simulink model "BaseEngineController_LS_112"  (Simulink 7.7)
settings: Solver=FixedStepDiscrete  StartTime=0.0  StopTime=10.0  RelTol=1e-3
PreLoadFcn:
  | try, eval([bdroot '_setup']); catch, eval('model_setup', ''); end
InitFcn:
  | try, eval([bdroot '_setup']); catch, eval('model_setup', ''); end
undefined symbols (not defined in the file): ECM, H1, H2, High, motohawk_build_version, motohawk_trunc_name, motohawk_vardec_config_group, motohawk_vardec_path, True, xD
libraries: MotoHawk_lib x1417, motohawk_control_primitives_lib x183, motohawk_engine_lib x32, simulink x21, motohawk_annotations_lib x9, AutoDoc_lib x8, simulink_extras x4, motohawk_ccp_examples_lib x1, motohawk_control_primitives_motoshare_lib x1
(part 16 of 27)

== system BaseEngineController_LS_112/Foreground/Control/VirtualSensors/AirCalcs/Speed Density - MAP Referenced - Adaptive ==
  note: mdot = rho V A = rho Q = (p/RT) (ve Vcyl) (Neng Ncyl / 60 NRPC )
  BARO [kPa] : Inport
  MAP [kPa] : Inport  Port=2
  RPM : Inport  Port=3
  IAT [C] : Inport  Port=4
  MAF_Sensor [g/s] : Inport  Port=5
  IAT17Idx : Inport  Port=6
  RPMIdx : Inport  Port=7
  SSEngOpr [bool] : Inport  Port=8
  ECT09Idx : Inport  Port=9
  ECT [C] : Inport  Port=10
  TimeAfterRun [S] : Inport  Port=11
  EngState : Inport  Port=12
  Adapt VolEff Map : Subsystem
  C to K1 : Subsystem
      mask Display: disp('to')
  Compare To Constant : simulink/Logic and Bit Operations/Compare To Constant  SystemSampleTime=-1  relop===  const=3  LogicOutDataTypeMode=boolean
  Cylinder Swept Volume [cm3]1 : MotoHawk_lib/Data Storage Blocks/motohawk_data_def  nam='CylSweptVol'  container_nam=''  data=373.5  typ=double  struct_nam='MyStruct'  storage=Constant  outputRef=off  use_vardec=on  window=Calibration  read_level=1  write_level=1  ovr_cals=on  view_as=Number  enum_struct={'Disabled', 'Enabled'}  vector_style=Wide Row  use_help_units=off  help='Cylinder swept volume for a single cylinder.'  units='cm3'  use_header_enum=off  row_header_enum={}  col_header_enum={}  use_min_max=off  min_val=0  max_val=inf  use_precision=on  precision=''  gain=1  offset=0  exp=1  use_mototune_group=on  mototune_group=motohawk_vardec_path(gcb)  eval_name=CylSweptVol  data_stores=motohawk_sfun_data_def_data_stores  struct_instances=motohawk_sfun_data_def_struct_instances  vardecs=motohawk_sfun_data_def_vardecs
  Cylinder Swept Volume [cm3] : MotoHawk_lib/Data Storage Blocks/motohawk_data_read  source=Lookup By Name  structure=Scalar  operation=Read scalar from location by index  sz_vec=-1  sz_row=-1  sz_col=-1  typ=double  nam='CylSweptVol'  checkNull=on  struct_inst_name='Struct1'  struct_nam='MyStruct'
  Data Type Conversion : DataTypeConversion  SaturateOnIntegerOverflow=on  RndMeth=Zero
  Gas Const [J/kg-K] : Constant  Value=287  OutDataTypeStr=Inherit: Inherit via back propagation
  Logical Operator : Logic  Inputs=6
  Logical Operator1 : Logic  Operator=NOT  AllPortsSameDT=off  OutDataTypeStr=boolean
  Model Air Mass Flow Rate : Product  Inputs=**  SaturateOnIntegerOverflow=on  InputSameDT=on  OutDataTypeStr=Inherit: Same as first input
  Multiport Switch : MultiPortSwitch  DataPortOrder=Zero-based contiguous  Inputs=2  zeroidx=on  SaturateOnIntegerOverflow=on  InputSameDT=on
  Nominal Air Flow Rate : Product  Inputs=******///  SaturateOnIntegerOverflow=on  InputSameDT=on  OutDataTypeStr=Inherit: Same as first input
  Number of Combustion Events Per Revolution : MotoHawk_lib/Data Storage Blocks/motohawk_data_read  source=Lookup By Name  structure=Scalar  operation=Read scalar from location by index  sz_vec=-1  sz_row=-1  sz_col=-1  typ=uint8  nam='CombEventsPerRev'  checkNull=on  struct_inst_name='Struct1'  struct_nam='MyStruct'
  Number of Combustion Events Per Revolution1 : MotoHawk_lib/Data Storage Blocks/motohawk_data_def  nam='CombEventsPerRev'  container_nam=''  data=1  typ=uint8  struct_nam='MyStruct'  storage=Constant  outputRef=off  use_vardec=on  window=Calibration  read_level=1  write_level=1  ovr_cals=on  view_as=Number  enum_struct={'Disabled', 'Enabled'}  vector_style=Wide Row  use_help_units=on  help='Number of conbustion events per engine revolution. For example, for a four-stroke, eight cylinder engine the value would be 4.'  units=''  use_header_enum=off  row_header_enum={}  col_header_enum={}  use_min_max=on  min_val=.5  max_val=inf  use_precision=off  precision=''  gain=1  offset=0  exp=1  use_mototune_group=on  mototune_group=motohawk_vardec_path(gcb)  eval_name=CombEventsPerRev  data_stores=motohawk_sfun_data_def_data_stores  struct_instances=motohawk_sfun_data_def_struct_instances  vardecs=motohawk_sfun_data_def_vardecs
  Relational Operator1 : RelationalOperator  InputSameDT=on
  Relational Operator2 : RelationalOperator  InputSameDT=on
  Sum : Sum  Inputs=|++
  Units Equivalency Factor : Constant  Value=60  OutDataTypeStr=Inherit: Inherit via back propagation
  motohawk_calibration : MotoHawk_lib/Calibration & Probing Blocks/motohawk_calibration  nam='VEAdaptEnable'  val=0  storage=Calibration  show_more=on  name_source=Use Parameter  data_type=boolean  read_level=1  write_level=1  ovr_cals=on  view_as=Enumeration  enum_struct={'Disabled', 'Enabled'}  vector_style=Wide Row  use_help_units=on  help='Determines whether the Volumetric Efficiency map will be adapted using the MAF sensor'  units='bool'  use_header_enum=off  row_header_enum={}  col_header_enum={}  use_min_max=off  min_val=-inf  max_val=inf  use_precision=off  precision=''  gain=1  offset=0  exp=1  use_mototune_group=on  mototune_group=motohawk_vardec_path(gcb)
  motohawk_calibration1 : MotoHawk_lib/Calibration & Probing Blocks/motohawk_calibration  nam='MAF_Source'  val=0  storage=Calibration  show_more=on  name_source=Use Parameter  data_type=uint8  read_level=1  write_level=1  ovr_cals=on  view_as=Enumeration  enum_struct={'Model from MAP', 'Use MAF sensor directly'}  vector_style=Wide Row  use_help_units=on  help='Selects the source for the fueling algorithm'  units=''  use_header_enum=off  row_header_enum={}  col_header_enum={}  use_min_max=off  min_val=-inf  max_val=inf  use_precision=off  precision=''  gain=1  offset=0  exp=1  use_mototune_group=on  mototune_group=motohawk_vardec_path(gcb)
  motohawk_calibration2 : MotoHawk_lib/Calibration & Probing Blocks/motohawk_calibration  nam='VEAdaptTemp'  val=60  storage=Calibration  show_more=on  name_source=Use Parameter  data_type=Inherit from 'Default Value'  read_level=1  write_level=1  ovr_cals=on  view_as=Number  enum_struct={'Disabled', 'Enabled'}  vector_style=Wide Row  use_help_units=on  help='Engine Coolant Temp Must be higher than this to Adapt VE'  units='degC'  use_header_enum=off  row_header_enum={}  col_header_enum={}  use_min_max=on  min_val=-40  max_val=200  use_precision=off  precision=''  gain=1  offset=0  exp=1  use_mototune_group=on  mototune_group=motohawk_vardec_path(gcb)
  motohawk_calibration3 : MotoHawk_lib/Calibration & Probing Blocks/motohawk_calibration  nam='VEAdaptTime'  val=60  storage=Calibration  show_more=on  name_source=Use Parameter  data_type=Inherit from 'Default Value'  read_level=1  write_level=1  ovr_cals=on  view_as=Number  enum_struct={'Disabled', 'Enabled'}  vector_style=Wide Row  use_help_units=on  help='Engine Run Time must be greater than this to Adapt VE'  units='sec'  use_header_enum=off  row_header_enum={}  col_header_enum={}  use_min_max=on  min_val=0  max_val=200  use_precision=off  precision=''  gain=1  offset=0  exp=1  use_mototune_group=on  mototune_group=motohawk_vardec_path(gcb)
  motohawk_fault_action1 : MotoHawk_lib/Fault Management Blocks/motohawk_fault_action  nam='DisableVEAdapt'  output_status=on  eval_nam=DisableVEAdapt
  motohawk_interpolation_1d1 : MotoHawk_lib/Lookup Tables/motohawk_interpolation_1d  nam='VEBaroCorr'  table_data=[1 1 1 1 1 1 1 1 1]  show_more=on  data_type=Inherit from 'Table Data'  storage=NonAdaptive  read_level=1  write_level=1  ovr_cals=on  use_help=on  help='Vol Eff compensation based on BARO.'  units=''  use_min_max=on  min_val=-inf  max_val=inf  use_precision=on  precision=''  gain=1  offset=0  exp=1  use_links=off  prelookup_block=''  output_name=''  use_mototune_group=on  mototune_group=motohawk_vardec_path(gcb)
  motohawk_interpolation_2d : MotoHawk_lib/Lookup Tables/motohawk_interpolation_2d  nam='VolEff'  table_data=ones(17)  show_more=on  data_type=Inherit from 'Table Data'  storage=NonAdaptive  read_level=1  write_level=1  ovr_cals=on  use_help=on  help='Volumetric efficiency table for speed density mode'  units='%'  use_min_max=on  min_val=0  max_val=1000  use_precision=on  precision=''  gain=1  offset=0  exp=1  use_links=on  row_prelookup_block=''  col_prelookup_block=''  output_name=''  use_mototune_group=on  mototune_group=motohawk_vardec_path(gcb)
  motohawk_interpolation_2d1 : MotoHawk_lib/Lookup Tables/motohawk_interpolation_2d  nam='VETempCorr'  table_data=ones(17,9)  show_more=on  data_type=Inherit from 'Table Data'  storage=NonAdaptive  read_level=1  write_level=1  ovr_cals=on  use_help=on  help=''  units='%'  use_min_max=off  min_val=-inf  max_val=inf  use_precision=off  precision=''  gain=1  offset=0  exp=1  use_links=off  row_prelookup_block=''  col_prelookup_block=''  output_name=''  use_mototune_group=off  mototune_group=motohawk_vardec_path(gcb)
  motohawk_interpolation_2d2 : MotoHawk_lib/Lookup Tables/motohawk_interpolation_2d  nam='VolEffAdapt'  table_data=ones(17)  show_more=on  data_type=Inherit from 'Table Data'  storage=Adaptive - NonVolatile  read_level=1  write_level=1  ovr_cals=on  use_help=on  help='Volumetric efficiency adapt table'  units='%'  use_min_max=on  min_val=-1000  max_val=1000  use_precision=on  precision=''  gain=1  offset=0  exp=1  use_links=on  row_prelookup_block=''  col_prelookup_block=''  output_name=''  use_mototune_group=on  mototune_group=motohawk_vardec_path(gcb)
  motohawk_prelookup1 : MotoHawk_lib/Lookup Tables/motohawk_prelookup  nam='BARO09'  breakpoint_data=[60 70 75 80 85 90 95 98 100]  show_more=on  data_type=Inherit from 'Table Data'  storage=Constant  read_level=1  write_level=1  ovr_cals=on  use_help=on  help=''  units=''  use_min_max=off  min_val=-inf  max_val=inf  use_precision=on  precision=''  gain=1  offset=0  exp=1  use_links=on  input_name='BARO'  use_mototune_group=on  mototune_group=motohawk_vardec_path(gcb)
  motohawk_prelookup2 : MotoHawk_lib/Lookup Tables/motohawk_prelookup  nam='VEMap'  breakpoint_data=[1:17]  show_more=on  data_type=Inherit from 'Table Data'  storage=Constant  read_level=1  write_level=1  ovr_cals=on  use_help=on  help='Index of MAP for VE calculations'  units='kPa'  use_min_max=off  min_val=-inf  max_val=inf  use_precision=on  precision=''  gain=1  offset=0  exp=1  use_links=off  input_name=''  use_mototune_group=on  mototune_group=motohawk_vardec_path(gcb)
  motohawk_probe : MotoHawk_lib/Calibration & Probing Blocks/motohawk_probe  nam='VEModelMAF'  show_more=on  name_source=Use Parameter  read_level=1  view_as=Number  enum_struct={'Disabled', 'Enabled'}  vector_style=Wide Row  use_help_units=on  help='Air Mass Flow Rate - Port Total'  units='g/s'  use_header_enum=off  row_header_enum={}  col_header_enum={}  use_precision=off  precision=''  gain=1  offset=0  exp=1  use_mototune_group=on  mototune_group=motohawk_vardec_path(gcb)
  motohawk_probe1 : MotoHawk_lib/Calibration & Probing Blocks/motohawk_probe  nam='VEIdealMAF'  show_more=on  name_source=Use Parameter  read_level=1  view_as=Number  enum_struct={'Disabled', 'Enabled'}  vector_style=Wide Row  use_help_units=on  help='Air Mass Flow Rate - ideal'  units='g/s'  use_header_enum=off  row_header_enum={}  col_header_enum={}  use_precision=off  precision=''  gain=1  offset=0  exp=1  use_mototune_group=on  mototune_group=motohawk_vardec_path(gcb)
  motohawk_probe3 : MotoHawk_lib/Calibration & Probing Blocks/motohawk_probe  nam='MAFFinal'  show_more=on  name_source=Use Parameter  read_level=1  view_as=Number  enum_struct={'Disabled', 'Enabled'}  vector_style=Wide Row  use_help_units=on  help='Air mass flow rate at the intake manifold - Used by the fueling algorithm'  units='g/s'  use_header_enum=off  row_header_enum={}  col_header_enum={}  use_precision=off  precision=''  gain=1  offset=0  exp=1  use_mototune_group=on  mototune_group=motohawk_vardec_path(gcb)
  motohawk_probe4 : MotoHawk_lib/Calibration & Probing Blocks/motohawk_probe  nam='VEAdapting'  show_more=on  name_source=Use Parameter  read_level=1  view_as=Enumeration  enum_struct={'Not adapting', 'Adapting'}  vector_style=Wide Row  use_help_units=on  help='Indicates whether the volumetric efficiency map is currently being adjusted'  units=''  use_header_enum=off  row_header_enum={}  col_header_enum={}  use_precision=off  precision=''  gain=1  offset=0  exp=1  use_mototune_group=on  mototune_group=motohawk_vardec_path(gcb)
  motohawk_probe5 : MotoHawk_lib/Calibration & Probing Blocks/motohawk_probe  nam='VEFin'  show_more=on  name_source=Use Parameter  read_level=1  view_as=Number  enum_struct={'Disabled', 'Enabled'}  vector_style=Wide Row  use_help_units=on  help='Final volumentric efficiency after adapt table'  units='g/s'  use_header_enum=off  row_header_enum={}  col_header_enum={}  use_precision=off  precision=''  gain=1  offset=0  exp=1  use_mototune_group=on  mototune_group=motohawk_vardec_path(gcb)
  motohawk_probe6 : MotoHawk_lib/Calibration & Probing Blocks/motohawk_probe  nam='VEAdaptAmnt'  show_more=on  name_source=Use Parameter  read_level=1  view_as=Number  enum_struct={'Disabled', 'Enabled'}  vector_style=Wide Row  use_help_units=on  help='Volumetric efficiency adapt amount at the given speed and load'  units='%'  use_header_enum=off  row_header_enum={}  col_header_enum={}  use_precision=off  precision=''  gain=1  offset=0  exp=1  use_mototune_group=on  mototune_group=motohawk_vardec_path(gcb)
  MAF [g/s] : Outport
  wires:
  motohawk_calibration1/1 -> Multiport Switch/1
  Multiport Switch/1 -> motohawk_probe3/1, MAF [g/s]/1
  MAF_Sensor [g/s]/1 -> Multiport Switch/3, Adapt VolEff Map/1(MAFSens)
  RPMIdx/1 -> motohawk_interpolation_2d/2, motohawk_interpolation_2d2/2
  motohawk_prelookup2/1 -> motohawk_interpolation_2d/1, motohawk_interpolation_2d2/1
  Model Air Mass Flow Rate/1 -> motohawk_probe/1, Multiport Switch/2, Adapt VolEff Map/2(MAFSpdDensity)
  IAT [C]/1 -> C to K1/1(C)
  RPM/1 -> Nominal Air Flow Rate/1
  BARO [kPa]/1 -> motohawk_prelookup1/1
  MAP [kPa]/1 -> Nominal Air Flow Rate/2, motohawk_prelookup2/1
  motohawk_interpolation_2d1/1 -> Nominal Air Flow Rate/4
  Cylinder Swept Volume [cm3]/1 -> Nominal Air Flow Rate/5
  Number of Combustion Events Per Revolution/1 -> Data Type Conversion/1
  C to K1/1(K) -> Nominal Air Flow Rate/7
  Units Equivalency Factor/1 -> Nominal Air Flow Rate/8
  Gas Const [J/kg-K]/1 -> Nominal Air Flow Rate/9
  Nominal Air Flow Rate/1 -> Model Air Mass Flow Rate/2, motohawk_probe1/1
  Data Type Conversion/1 -> Nominal Air Flow Rate/6
  motohawk_prelookup1/1 -> motohawk_interpolation_1d1/1
  motohawk_interpolation_1d1/1 -> Nominal Air Flow Rate/3
  IAT17Idx/1 -> motohawk_interpolation_2d1/1
  ECT09Idx/1 -> motohawk_interpolation_2d1/2
  motohawk_fault_action1/1 -> Logical Operator1/1
  EngState/1 -> Compare To Constant/1
  Compare To Constant/1 -> Logical Operator/1
  Logical Operator1/1 -> Logical Operator/2
  SSEngOpr [bool]/1 -> Logical Operator/3
  ECT [C]/1 -> Relational Operator1/1
  Relational Operator1/1 -> Logical Operator/4
  Relational Operator2/1 -> Logical Operator/5
  motohawk_calibration2/1 -> Relational Operator1/2
  TimeAfterRun [S]/1 -> Relational Operator2/1
  motohawk_calibration3/1 -> Relational Operator2/2
  Logical Operator/1 -> Adapt VolEff Map/Enable, motohawk_probe4/1
  motohawk_calibration/1 -> Logical Operator/6
  motohawk_interpolation_2d/1 -> Sum/1
  motohawk_interpolation_2d2/1 -> Sum/2, motohawk_probe6/1
  Sum/1 -> Model Air Mass Flow Rate/1, Adapt VolEff Map/3(VE), motohawk_probe5/1

== system BaseEngineController_LS_112/Foreground/Control/VirtualSensors/FuelLevel/FuelLevelWrite ==
  FuelLevelFilt : Inport
  Enable : EnablePort
  motohawk_data_write : MotoHawk_lib/Data Storage Blocks/motohawk_data_write  source=Lookup By Name  structure=Scalar  operation=Write entire data structure at once  sz_vec=9  sz_row=2  sz_col=9  typ=double  nam='FuelLvl_NVM'  checkNull=on  write_read_only=off  struct_inst_name=''  struct_name='MyStruct'
  wires:
  FuelLevelFilt/1 -> motohawk_data_write/1

== system BaseEngineController_LS_112/Foreground/Control/VirtualSensors/FuelLevel/RefuelEvent ==
  FuelRaw : Inport
  TimeSinceKeyOn : Inport  Port=2
  Logical Operator : Logic  AllPortsSameDT=off  OutDataTypeStr=boolean
  Relational Operator : RelationalOperator  OutDataTypeStr=boolean
  Relational Operator1 : RelationalOperator  OutDataTypeStr=boolean
  Rising Edge : motohawk_control_primitives_lib/Rising Edge  SystemSampleTime=-1
  Sum : Sum  Inputs=|+-
  motohawk_calibration1 : MotoHawk_lib/Calibration & Probing Blocks/motohawk_calibration  nam='FuelLevl_KeyUpDiff'  val=5  storage=Calibration  show_more=on  name_source=Use Parameter  data_type=Inherit from 'Default Value'  read_level=1  write_level=1  ovr_cals=on  view_as=Number  enum_struct={'Disabled', 'Enabled'}  vector_style=Wide Row  use_help_units=on  help='Fuel level key up different for refuel event'  units='%'  use_header_enum=off  row_header_enum={}  col_header_enum={}  use_min_max=on  min_val=0  max_val=inf  use_precision=off  precision=''  gain=1  offset=0  exp=1  use_mototune_group=off  mototune_group=motohawk_vardec_path(gcb)
  motohawk_calibration10 : MotoHawk_lib/Calibration & Probing Blocks/motohawk_calibration  nam='FuelLevel_KeyUpDelay'  val=.2  storage=Calibration  show_more=on  name_source=Use Parameter  data_type=Inherit from 'Default Value'  read_level=1  write_level=1  ovr_cals=on  view_as=Number  enum_struct={'Disabled', 'Enabled'}  vector_style=Wide Row  use_help_units=on  help='Fuel level time from key on delay'  units='sec'  use_header_enum=off  row_header_enum={}  col_header_enum={}  use_min_max=on  min_val=0  max_val=inf  use_precision=off  precision=''  gain=1  offset=0  exp=1  use_mototune_group=off  mototune_group=motohawk_vardec_path(gcb)
  motohawk_data_read : MotoHawk_lib/Data Storage Blocks/motohawk_data_read  source=Lookup By Name  structure=Scalar  operation=Read scalar from location by index  sz_vec=4  sz_row=2  sz_col=3  typ=double  nam='FuelLvl_NVM'  checkNull=on  struct_inst_name='MyData'  struct_nam='MyStruct'
  motohawk_probe : MotoHawk_lib/Calibration & Probing Blocks/motohawk_probe  nam='FuelLevel_RefuelEvent'  show_more=off  name_source=Use Parameter  read_level=1  view_as=Number  enum_struct={'Disabled', 'Enabled'}  vector_style=Wide Row  use_help_units=off  help=''  units=''  use_header_enum=off  row_header_enum={}  col_header_enum={}  use_precision=off  precision=''  gain=1  offset=0  exp=1  use_mototune_group=off  mototune_group=motohawk_vardec_path(gcb)
  RefuelEvent : Outport
  RefuelEventDR : Outport  Port=2
  wires:
  TimeSinceKeyOn/1 -> Relational Operator/1
  motohawk_calibration10/1 -> Relational Operator/2
  Relational Operator/1 -> RefuelEventDR/1, Logical Operator/2
  FuelRaw/1 -> Sum/1
  motohawk_data_read/1 -> Sum/2
  Sum/1 -> Relational Operator1/1
  motohawk_calibration1/1 -> Relational Operator1/2
  Relational Operator1/1 -> Logical Operator/1
  Logical Operator/1 -> Rising Edge/1
  Rising Edge/1 -> RefuelEvent/1, motohawk_probe/1

== system BaseEngineController_LS_112/Foreground/Control/VirtualSensors/LoadBasedCalcs/Engine Steady-State Flag ==
  Load : Inport
  RPM : Inport  Port=2
  Abs : Abs  SaturateOnIntegerOverflow=on
  Abs1 : Abs  SaturateOnIntegerOverflow=on
  Constant : Constant  Value=0  OutDataTypeStr=Inherit: Inherit via back propagation
  Inc_DecFilterSelect1 : Subsystem  AncestorBlock=motohawk_control_primitives_lib/Inc_DecFilterSelect1  mask{nam='SSRPM', grp_dis=group, grp_cal=motohawk_vardec_config_group(group)}
      mask prompts: nam "Signal Name"; grp_dis "MotoTune Display Group"; grp_cal "MotoTune Calibration Group"
      mask Display:
      | patch([0 0 1 1], [0 0.075 0.075 0], [230/255 0/255 0/255])
      | patch([0 0 1 1], [0.025 0.05 0.05 0.025], [150/255 0/255 0/255])
      | patch([0 0 1 1], [0 0.025 0.025 0], [0/255 0/255 0/255])
      | 
      | disp('Increasing/Decreasing\nFiler Select');
  Inc_DecFilterSelect3 : Subsystem  AncestorBlock=motohawk_control_primitives_lib/Inc_DecFilterSelect1  mask{nam='SSLoad', grp_dis=group, grp_cal=motohawk_vardec_config_group(group)}
      mask prompts: nam "Signal Name"; grp_dis "MotoTune Display Group"; grp_cal "MotoTune Calibration Group"
      mask Display:
      | patch([0 0 1 1], [0 0.075 0.075 0], [230/255 0/255 0/255])
      | patch([0 0 1 1], [0.025 0.05 0.05 0.025], [150/255 0/255 0/255])
      | patch([0 0 1 1], [0 0.025 0.025 0], [0/255 0/255 0/255])
      | 
      | disp('Increasing/Decreasing\nFiler Select');
  Logical Operator : Logic  Inputs=3
  Relational Operator : RelationalOperator  Operator=<=  InputSameDT=on
  Relational Operator1 : RelationalOperator  Operator=<=  InputSameDT=on
  Relational Operator2 : RelationalOperator  Operator=>  ZeroCross=off  InputSameDT=on
  Steady-state RPM Tolerance [RPM] : MotoHawk_lib/Calibration & Probing Blocks/motohawk_calibration  nam='SSRPMTol'  val=600  storage=Calibration  show_more=on  name_source=Use Parameter  data_type=Inherit from 'Default Value'  read_level=1  write_level=1  ovr_cals=on  view_as=Number  enum_struct={'Disabled', 'Enabled'}  vector_style=Wide Row  use_help_units=on  help='Steady-State RPM Tolerance'  units='RPM'  use_header_enum=off  row_header_enum={}  col_header_enum={}  use_min_max=off  min_val=-inf  max_val=inf  use_precision=off  precision=''  gain=1  offset=0  exp=1  use_mototune_group=on  mototune_group=motohawk_vardec_path(gcb)
  Steady-state Torque Tolerance [N.m] : MotoHawk_lib/Calibration & Probing Blocks/motohawk_calibration  nam='SSLoadTol'  val=100  storage=Calibration  show_more=on  name_source=Use Parameter  data_type=Inherit from 'Default Value'  read_level=1  write_level=1  ovr_cals=on  view_as=Number  enum_struct={'Disabled', 'Enabled'}  vector_style=Wide Row  use_help_units=on  help='Steady-State Load Tolerance'  units=''  use_header_enum=off  row_header_enum={}  col_header_enum={}  use_min_max=off  min_val=-inf  max_val=inf  use_precision=off  precision=''  gain=1  offset=0  exp=1  use_mototune_group=on  mototune_group=motohawk_vardec_path(gcb)
  Sum : Sum  Inputs=+-|  SaturateOnIntegerOverflow=on  InputSameDT=on  OutDataTypeStr=Inherit: Same as first input
  Sum1 : Sum  Inputs=+-|  SaturateOnIntegerOverflow=on  InputSameDT=on  OutDataTypeStr=Inherit: Same as first input
  motohawk_probe : MotoHawk_lib/Calibration & Probing Blocks/motohawk_probe  nam='SSEngOpr'  show_more=on  name_source=Use Parameter  read_level=1  view_as=Enumeration  enum_struct={'Transient', 'Steady'}  vector_style=Wide Row  use_help_units=on  help='Steady-State Engine Operation'  units=''  use_header_enum=off  row_header_enum={}  col_header_enum={}  use_precision=off  precision=''  gain=1  offset=0  exp=1  use_mototune_group=on  mototune_group=motohawk_vardec_path(gcb)
  SSEngOpr [bool] : Outport
  wires:
  Steady-state RPM Tolerance [RPM]/1 -> Relational Operator1/2
  Steady-state Torque Tolerance [N.m]/1 -> Relational Operator/2
  Inc_DecFilterSelect1/1(Out) -> Sum1/2
  Logical Operator/1 -> SSEngOpr [bool]/1, motohawk_probe/1
  Abs1/1 -> Relational Operator1/1
  Sum1/1 -> Abs1/1
  Abs/1 -> Relational Operator/1
  Sum/1 -> Abs/1
  Inc_DecFilterSelect3/1(Out) -> Sum/2
  RPM/1 -> Sum1/1, Relational Operator2/1, Inc_DecFilterSelect1/1(In)
  Load/1 -> Sum/1, Inc_DecFilterSelect3/1(In)
  Relational Operator1/1 -> Logical Operator/1
  Relational Operator/1 -> Logical Operator/3
  Relational Operator2/1 -> Logical Operator/2
  Constant/1 -> Relational Operator2/2

== system BaseEngineController_LS_112/Foreground/Control/VirtualSensors/Raw Indexes/ACPres Index ==
  ACPres : Inport
  motohawk_prelookup : MotoHawk_lib/Lookup Tables/motohawk_prelookup  nam='ACPres05'  breakpoint_data=[1500 1750 2000 2250 2500]  show_more=on  data_type=Inherit from 'Table Data'  storage=Constant  read_level=1  write_level=1  ovr_cals=on  use_help=on  help='Index of AC system high side pressure'  units='kPa'  use_min_max=on  min_val=-150  max_val=10000  use_precision=on  precision=''  gain=1  offset=0  exp=1  use_links=off  input_name=''  use_mototune_group=on  mototune_group=motohawk_vardec_path(gcb)
  motohawk_prelookup1 : MotoHawk_lib/Lookup Tables/motohawk_prelookup  nam='ACPres07'  breakpoint_data=[1500 1750 2000 2250 2500 2500 2500]  show_more=on  data_type=Inherit from 'Table Data'  storage=Constant  read_level=1  write_level=1  ovr_cals=on  use_help=on  help='Index of AC system high side pressure'  units='kPa'  use_min_max=on  min_val=-150  max_val=10000  use_precision=on  precision=''  gain=1  offset=0  exp=1  use_links=off  input_name=''  use_mototune_group=on  mototune_group=motohawk_vardec_path(gcb)
  ACPres05Idx : Outport
  ACPres07Idx : Outport  Port=2
  wires:
  ACPres/1 -> motohawk_prelookup/1, motohawk_prelookup1/1
  motohawk_prelookup/1 -> ACPres05Idx/1
  motohawk_prelookup1/1 -> ACPres07Idx/1

== system BaseEngineController_LS_112/Foreground/Control/VirtualSensors/Raw Indexes/CAT Index ==
  CAT : Inport
  motohawk_prelookup : MotoHawk_lib/Lookup Tables/motohawk_prelookup  nam='CAT05'  breakpoint_data=[-40:35:100]  show_more=on  data_type=Inherit from 'Table Data'  storage=Constant  read_level=1  write_level=1  ovr_cals=on  use_help=on  help='Index of charge air temperature'  units='degC'  use_min_max=on  min_val=-40  max_val=300  use_precision=on  precision=''  gain=1  offset=0  exp=1  use_links=off  input_name=''  use_mototune_group=on  mototune_group=motohawk_vardec_path(gcb)
  CAT05Idx : Outport
  wires:
  CAT/1 -> motohawk_prelookup/1
  motohawk_prelookup/1 -> CAT05Idx/1

== system BaseEngineController_LS_112/Foreground/Control/VirtualSensors/Raw Indexes/ECT Index ==
  ECT : Inport
  motohawk_prelookup : MotoHawk_lib/Lookup Tables/motohawk_prelookup  nam='ECT05'  breakpoint_data=[-20 0 20 40 80]  show_more=on  data_type=Inherit from 'Table Data'  storage=Constant  read_level=1  write_level=1  ovr_cals=on  use_help=on  help='Idex of ECT'  units='degC'  use_min_max=on  min_val=-40  max_val=200  use_precision=on  precision=''  gain=1  offset=0  exp=1  use_links=off  input_name=''  use_mototune_group=on  mototune_group=motohawk_vardec_path(gcb)
  motohawk_prelookup1 : MotoHawk_lib/Lookup Tables/motohawk_prelookup  nam='ECT09'  breakpoint_data=[-40 -20 0 10 20 40 80 100 120]  show_more=on  data_type=Inherit from 'Table Data'  storage=Constant  read_level=1  write_level=1  ovr_cals=on  use_help=on  help='Index of ECT'  units='degC'  use_min_max=on  min_val=-40  max_val=200  use_precision=on  precision=''  gain=1  offset=0  exp=1  use_links=off  input_name=''  use_mototune_group=on  mototune_group=motohawk_vardec_path(gcb)
  motohawk_prelookup2 : MotoHawk_lib/Lookup Tables/motohawk_prelookup  nam='ECT07'  breakpoint_data=[-40 -20 0 10 20 40 80]  show_more=on  data_type=Inherit from 'Table Data'  storage=Constant  read_level=1  write_level=1  ovr_cals=on  use_help=on  help='Index of ECT'  units='degC'  use_min_max=on  min_val=-40  max_val=200  use_precision=on  precision=''  gain=1  offset=0  exp=1  use_links=off  input_name=''  use_mototune_group=on  mototune_group=motohawk_vardec_path(gcb)
  ECT05Idx : Outport
  ECT07Idx : Outport  Port=2
  ECT09Idx : Outport  Port=3
  wires:
  ECT/1 -> motohawk_prelookup/1, motohawk_prelookup1/1, motohawk_prelookup2/1
  motohawk_prelookup/1 -> ECT05Idx/1
  motohawk_prelookup1/1 -> ECT09Idx/1
  motohawk_prelookup2/1 -> ECT07Idx/1

== system BaseEngineController_LS_112/Foreground/Control/VirtualSensors/Raw Indexes/IAT Indexes ==
  IAT : Inport
  motohawk_prelookup : MotoHawk_lib/Lookup Tables/motohawk_prelookup  nam='IAT05'  breakpoint_data=[-20 -5 10 30 60]  show_more=on  data_type=Inherit from 'Table Data'  storage=Constant  read_level=1  write_level=1  ovr_cals=on  use_help=on  help='Index of IAT'  units='degC'  use_min_max=on  min_val=-40  max_val=300  use_precision=on  precision=''  gain=1  offset=0  exp=1  use_links=off  input_name=''  use_mototune_group=on  mototune_group=motohawk_vardec_path(gcb)
  motohawk_prelookup1 : MotoHawk_lib/Lookup Tables/motohawk_prelookup  nam='IAT07'  breakpoint_data=[-20:((60+20)/(7-1)):60]  show_more=on  data_type=Inherit from 'Table Data'  storage=Constant  read_level=1  write_level=1  ovr_cals=on  use_help=on  help='Index of IAT'  units='degC'  use_min_max=on  min_val=-40  max_val=300  use_precision=on  precision=''  gain=1  offset=0  exp=1  use_links=off  input_name=''  use_mototune_group=on  mototune_group=motohawk_vardec_path(gcb)
  motohawk_prelookup2 : MotoHawk_lib/Lookup Tables/motohawk_prelookup  nam='IAT17'  breakpoint_data=[-20:((60+20)/(17-1)):60]  show_more=on  data_type=Inherit from 'Table Data'  storage=Constant  read_level=1  write_level=1  ovr_cals=on  use_help=on  help='Index of IAT'  units='degC'  use_min_max=on  min_val=-40  max_val=300  use_precision=on  precision=''  gain=1  offset=0  exp=1  use_links=off  input_name=''  use_mototune_group=on  mototune_group=motohawk_vardec_path(gcb)
  IAT05Idx : Outport
  IAT07Idx : Outport  Port=2
  IAT17Idx : Outport  Port=3
  wires:
  motohawk_prelookup/1 -> IAT05Idx/1
  IAT/1 -> motohawk_prelookup2/1, motohawk_prelookup/1, motohawk_prelookup1/1
  motohawk_prelookup2/1 -> IAT17Idx/1
  motohawk_prelookup1/1 -> IAT07Idx/1

== system BaseEngineController_LS_112/Foreground/Control/VirtualSensors/Raw Indexes/MAP Indexes ==
  MAP : Inport
  motohawk_prelookup : MotoHawk_lib/Lookup Tables/motohawk_prelookup  nam='MAP05'  breakpoint_data=[0:((110-0)/(5-1)):110]  show_more=on  data_type=Inherit from 'Table Data'  storage=Constant  read_level=1  write_level=1  ovr_cals=on  use_help=on  help='Index of MAP'  units='kPa'  use_min_max=on  min_val=0  max_val=1000  use_precision=on  precision=''  gain=1  offset=0  exp=1  use_links=off  input_name=''  use_mototune_group=on  mototune_group=motohawk_vardec_path(gcb)
  motohawk_prelookup1 : MotoHawk_lib/Lookup Tables/motohawk_prelookup  nam='MAP09'  breakpoint_data=[0:((110-0)/(9-1)):110]  show_more=on  data_type=Inherit from 'Table Data'  storage=Constant  read_level=1  write_level=1  ovr_cals=on  use_help=on  help='Index of MAP'  units='kPa'  use_min_max=on  min_val=0  max_val=1000  use_precision=on  precision=''  gain=1  offset=0  exp=1  use_links=off  input_name=''  use_mototune_group=on  mototune_group=motohawk_vardec_path(gcb)
  motohawk_prelookup5 : MotoHawk_lib/Lookup Tables/motohawk_prelookup  nam='MAP17'  breakpoint_data=[0:((110-0)/(17-1)):110]  show_more=on  data_type=Inherit from 'Table Data'  storage=Constant  read_level=1  write_level=1  ovr_cals=on  use_help=on  help='Index of MAP'  units='kPa'  use_min_max=on  min_val=0  max_val=1000  use_precision=on  precision=''  gain=1  offset=0  exp=1  use_links=off  input_name=''  use_mototune_group=on  mototune_group=motohawk_vardec_path(gcb)
  MAP05Idx : Outport
  MAP09Idx : Outport  Port=2
  MAP17Idx : Outport  Port=3
  wires:
  motohawk_prelookup/1 -> MAP05Idx/1
  motohawk_prelookup1/1 -> MAP09Idx/1
  MAP/1 -> motohawk_prelookup1/1, motohawk_prelookup5/1, motohawk_prelookup/1
  motohawk_prelookup5/1 -> MAP17Idx/1  "Indexes"

== system BaseEngineController_LS_112/Foreground/Control/VirtualSensors/Raw Indexes/OXY Index ==
  CAT : Inport
  motohawk_prelookup : MotoHawk_lib/Lookup Tables/motohawk_prelookup  nam='OXY05'  breakpoint_data=[0:22:100]  show_more=on  data_type=Inherit from 'Table Data'  storage=Constant  read_level=1  write_level=1  ovr_cals=on  use_help=on  help='Index of fuel oxygenation content'  units='%'  use_min_max=on  min_val=0  max_val=100  use_precision=on  precision=''  gain=1  offset=0  exp=1  use_links=off  input_name=''  use_mototune_group=on  mototune_group=motohawk_vardec_path(gcb)
  OXY05Idx : Outport
  wires:
  CAT/1 -> motohawk_prelookup/1
  motohawk_prelookup/1 -> OXY05Idx/1

== system BaseEngineController_LS_112/Foreground/Control/VirtualSensors/Raw Indexes/RPM Indexes ==
  RPM : Inport
  motohawk_prelookup : MotoHawk_lib/Lookup Tables/motohawk_prelookup  nam='RPM05'  breakpoint_data=[300:((4200-300)/(5-1)):4200]  show_more=on  data_type=Inherit from 'Table Data'  storage=Constant  read_level=1  write_level=1  ovr_cals=on  use_help=on  help='Index of RPM'  units='RPM'  use_min_max=on  min_val=0  max_val=14000  use_precision=on  precision=''  gain=1  offset=0  exp=1  use_links=off  input_name=''  use_mototune_group=on  mototune_group=motohawk_vardec_path(gcb)
  motohawk_prelookup1 : MotoHawk_lib/Lookup Tables/motohawk_prelookup  nam='RPM09'  breakpoint_data=[300:((4200-300)/(9-1)):4200]  show_more=on  data_type=Inherit from 'Table Data'  storage=Constant  read_level=1  write_level=1  ovr_cals=on  use_help=on  help='Index of RPM'  units='RPM'  use_min_max=on  min_val=0  max_val=14000  use_precision=on  precision=''  gain=1  offset=0  exp=1  use_links=off  input_name=''  use_mototune_group=on  mototune_group=motohawk_vardec_path(gcb)
  motohawk_prelookup5 : MotoHawk_lib/Lookup Tables/motohawk_prelookup  nam='RPM17'  breakpoint_data=[300:((4200-300)/(17-1)):4200]  show_more=on  data_type=Inherit from 'Table Data'  storage=Constant  read_level=1  write_level=1  ovr_cals=on  use_help=on  help='Index of RPM'  units='RPM'  use_min_max=on  min_val=0  max_val=14000  use_precision=on  precision=''  gain=1  offset=0  exp=1  use_links=off  input_name=''  use_mototune_group=on  mototune_group=motohawk_vardec_path(gcb)
  RPM05Idx : Outport
  RPM09Idx : Outport  Port=2
  RPM17Idx : Outport  Port=3
  wires:
  motohawk_prelookup/1 -> RPM05Idx/1
  motohawk_prelookup1/1 -> RPM09Idx/1
  RPM/1 -> motohawk_prelookup1/1, motohawk_prelookup5/1, motohawk_prelookup/1
  motohawk_prelookup5/1 -> RPM17Idx/1  "Indexes"

== system BaseEngineController_LS_112/Foreground/Control/VirtualSensors/Raw Indexes/SysVolt Index ==
  SysVolt : Inport
  motohawk_prelookup : MotoHawk_lib/Lookup Tables/motohawk_prelookup  nam='SysVolt09'  breakpoint_data=[7.99959 8.99966 9.99973 10.9998 11.99987 13.50046 14.00001 15.00008 16.000151]  show_more=on  data_type=Inherit from 'Table Data'  storage=Constant  read_level=1  write_level=1  ovr_cals=on  use_help=on  help='Index of system voltage'  units='Volts'  use_min_max=on  min_val=0  max_val=32  use_precision=on  precision=''  gain=1  offset=0  exp=1  use_links=off  input_name=''  use_mototune_group=on  mototune_group=motohawk_vardec_path(gcb)
  SysVolt09Idx : Outport
  wires:
  motohawk_prelookup/1 -> SysVolt09Idx/1
  SysVolt/1 -> motohawk_prelookup/1

== system BaseEngineController_LS_112/Foreground/Control/VirtualSensors/Raw Indexes/TPS Indexes ==
  TPSPcnt : Inport
  motohawk_prelookup2 : MotoHawk_lib/Lookup Tables/motohawk_prelookup  nam='TPS09'  breakpoint_data=[0:((100-0)/(9-1)):100]  show_more=on  data_type=Inherit from 'Table Data'  storage=Constant  read_level=1  write_level=1  ovr_cals=on  use_help=on  help='Index of TPS'  units='%'  use_min_max=on  min_val=0  max_val=100  use_precision=on  precision=''  gain=1  offset=0  exp=1  use_links=off  input_name=''  use_mototune_group=on  mototune_group=motohawk_vardec_path(gcb)
  TPS09Idx : Outport
  wires:
  TPSPcnt/1 -> motohawk_prelookup2/1
  motohawk_prelookup2/1 -> TPS09Idx/1

== system BaseEngineController_LS_112/Foreground/Control/VirtualSensors/Raw Indexes/VSPD Index ==
  VSPD : Inport
  motohawk_prelookup : MotoHawk_lib/Lookup Tables/motohawk_prelookup  nam='VSPD09'  breakpoint_data=[0:15:120]  show_more=on  data_type=Inherit from 'Table Data'  storage=Constant  read_level=1  write_level=1  ovr_cals=on  use_help=on  help='Index of VSPD'  units='MPH'  use_min_max=on  min_val=-100  max_val=200  use_precision=on  precision=''  gain=1  offset=0  exp=1  use_links=off  input_name=''  use_mototune_group=on  mototune_group=motohawk_vardec_path(gcb)
  motohawk_prelookup1 : MotoHawk_lib/Lookup Tables/motohawk_prelookup  nam='VSPD17'  breakpoint_data=[0:7.5:120]  show_more=on  data_type=Inherit from 'Table Data'  storage=Constant  read_level=1  write_level=1  ovr_cals=on  use_help=on  help='Index of VSPD'  units='MPH'  use_min_max=on  min_val=-100  max_val=200  use_precision=on  precision=''  gain=1  offset=0  exp=1  use_links=off  input_name=''  use_mototune_group=on  mototune_group=motohawk_vardec_path(gcb)
  motohawk_prelookup2 : MotoHawk_lib/Lookup Tables/motohawk_prelookup  nam='VSPD07'  breakpoint_data=[0:18:120]  show_more=on  data_type=Inherit from 'Table Data'  storage=Constant  read_level=1  write_level=1  ovr_cals=on  use_help=on  help='Index of VSPD'  units='MPH'  use_min_max=on  min_val=-100  max_val=200  use_precision=on  precision=''  gain=1  offset=0  exp=1  use_links=off  input_name=''  use_mototune_group=on  mototune_group=motohawk_vardec_path(gcb)
  VSPD09Idx : Outport
  VSPD07Idx : Outport  Port=2
  VSPD17Idx : Outport  Port=3
  wires:
  VSPD/1 -> motohawk_prelookup/1, motohawk_prelookup1/1, motohawk_prelookup2/1
  motohawk_prelookup/1 -> VSPD09Idx/1
  motohawk_prelookup1/1 -> VSPD17Idx/1
  motohawk_prelookup2/1 -> VSPD07Idx/1

== system BaseEngineController_LS_112/Foreground/Control/VirtualSensors/RawProcessed/APP  Sensor Arbitration1 ==
  note: Normally take TPS1
      | If TPS1 faulted, take TPS2
      | If both are faulted, take the larger
      | of the two to force ETC controller
      | to zero.
  note: Normally APP1
  APP1 : Inport
  APP2 : Inport  Port=2
  Abs : Abs  SaturateOnIntegerOverflow=on
  Logical Operator1 : Logic  Operator=OR  AllPortsSameDT=off
  Logical Operator4 : Logic  Operator=OR  AllPortsSameDT=off
  Logical Operator5 : Logic  Operator=OR  AllPortsSameDT=off
  Logical Operator6 : Logic  AllPortsSameDT=off
  MinMax : MinMax  Inputs=2
  Relational Operator3 : RelationalOperator  Operator=>  OutDataTypeStr=boolean
  Sum : Sum  Inputs=|+-  SaturateOnIntegerOverflow=on
  Switch1 : Switch  Threshold=1  SaturateOnIntegerOverflow=on
  Switch2 : Switch  Threshold=1  SaturateOnIntegerOverflow=on
  motohawk_calibration2 : MotoHawk_lib/Calibration & Probing Blocks/motohawk_calibration  nam='APP1_APP2_Max_Deviation'  val=100  storage=Calibration  show_more=on  name_source=Use Parameter  data_type=double  read_level=1  write_level=1  ovr_cals=on  view_as=Number  enum_struct={'Disabled', 'Enabled'}  vector_style=Wide Row  use_help_units=on  help='Specifies the maximum allowable deviation between the two sensors'  units='Percent'  use_header_enum=off  row_header_enum={}  col_header_enum={}  use_min_max=off  min_val=-inf  max_val=inf  use_precision=off  precision=''  gain=1  offset=0  exp=1  use_mototune_group=on  mototune_group=motohawk_vardec_path(gcb)
  motohawk_fault_def1 : MotoHawk_lib/Fault Management Blocks/motohawk_fault_def  nam='APP_Sensors_Conflict'  mode=Enabled  id=[]  x=25  y=50  input_suspected=on  indeterminate=off  increment_xy=on  downsample_count=1  ovr_cals=on  ovr_actions=on  show_actions=off  action1_name=''  action1_cond=(None)  action2_name=''  action2_cond=(None)  action3_name=''  action3_cond=(None)  action4_name=''  action4_cond=(None)
  motohawk_fault_status : MotoHawk_lib/Fault Management Blocks/motohawk_fault_status  source=Lookup By Name  nam='APP1RangeHigh'  status=Active
  motohawk_fault_status1 : MotoHawk_lib/Fault Management Blocks/motohawk_fault_status  source=Lookup By Name  nam='APP1RangeLow'  status=Active
  motohawk_fault_status2 : MotoHawk_lib/Fault Management Blocks/motohawk_fault_status  source=Lookup By Name  nam='APP2RangeLow'  status=Active
  motohawk_fault_status3 : MotoHawk_lib/Fault Management Blocks/motohawk_fault_status  source=Lookup By Name  nam='APP2RangeHigh'  status=Active
  motohawk_fault_status4 : MotoHawk_lib/Fault Management Blocks/motohawk_fault_status  source=Lookup By Name  nam='APP_Sensors_Conflict'  status=Active
  APP : Outport
  wires:
  Sum/1 -> Abs/1
  Abs/1 -> Relational Operator3/1
  motohawk_calibration2/1 -> Relational Operator3/2
  APP1/1 -> Sum/1, Switch1/3, MinMax/2
  APP2/1 -> Sum/2, Switch1/1, MinMax/1
  Relational Operator3/1 -> motohawk_fault_def1/1
  motohawk_fault_status/1 -> Logical Operator4/1
  motohawk_fault_status1/1 -> Logical Operator4/2
  motohawk_fault_status3/1 -> Logical Operator5/1
  motohawk_fault_status2/1 -> Logical Operator5/2
  Switch2/1 -> APP/1
  Logical Operator4/1 -> Switch1/2, Logical Operator6/1
  Logical Operator5/1 -> Logical Operator6/2
  Switch1/1 -> Switch2/3
  Logical Operator6/1 -> Logical Operator1/1  "Both Faulted"
  motohawk_fault_status4/1 -> Logical Operator1/2
  MinMax/1 -> Switch2/1
  Logical Operator1/1 -> Switch2/2

== system BaseEngineController_LS_112/Foreground/Control/VirtualSensors/RawProcessed/Base TPS Request ==
  APP Pcnt : Inport
  TPS_Idx : Inport  Port=2
  VSPD17Idx : Inport  Port=3
  First Order Low Pass : motohawk_control_primitives_lib/First Order Low Pass  SystemSampleTime=-1
  Merge : Merge
  MinMax : MinMax  Function=max  Inputs=2  SaturateOnIntegerOverflow=on  InputSameDT=on
  PassThrough1 : Subsystem  TreatAsAtomicUnit=on
  PassThrough2 : Subsystem  TreatAsAtomicUnit=on
  Product : Product  Inputs=*/  SaturateOnIntegerOverflow=on  InputSameDT=on  OutDataTypeStr=Inherit: Same as first input
  Relational Operator2 : RelationalOperator  Operator=>  OutDataTypeStr=boolean
  Relational Operator3 : RelationalOperator  Operator=<  OutDataTypeStr=boolean
  Unit Delay{1..4} (4 alike) : UnitDelay  SampleTime=-1
  Variable Rate Limiter : Subsystem  AncestorBlock=motohawk_control_primitives_lib_new/Variable Rate Limiter  mask(Variable Rate Limiter){}
      mask help: Variable Rate Limiter Block
      mask Display:
      | patch([0 0 1 1], [0 0.075 0.075 0], [230/255 0/255 0/255])
      | patch([0 0 1 1], [0.025 0.05 0.05 0.025], [150/255 0/255 0/255])
      | patch([0 0 1 1], [0 0.025 0.025 0], [0/255 0/255 0/255])
      | 
      | disp(['RATE \nLIMITER']);
  motohawk_calibration1 : MotoHawk_lib/Calibration & Probing Blocks/motohawk_calibration  nam='ETCReqIncFiltC'  val=0  storage=Calibration  show_more=on  name_source=Use Parameter  data_type=Inherit from 'Default Value'  read_level=1  write_level=1  ovr_cals=on  view_as=Number  enum_struct={'Disabled', 'Enabled'}  vector_style=Wide Row  use_help_units=on  help='Filter time constant for a decreasing ETC Request signal.'  units='sec'  use_header_enum=off  row_header_enum={}  col_header_enum={}  use_min_max=off  min_val=-inf  max_val=inf  use_precision=off  precision=''  gain=1  offset=0  exp=1  use_mototune_group=on  mototune_group=motohawk_vardec_path(gcb)
  motohawk_calibration2 : MotoHawk_lib/Calibration & Probing Blocks/motohawk_calibration  nam='ETCReqDecFiltC'  val=0  storage=Calibration  show_more=on  name_source=Use Parameter  data_type=Inherit from 'Default Value'  read_level=1  write_level=1  ovr_cals=on  view_as=Number  enum_struct={'Disabled', 'Enabled'}  vector_style=Wide Row  use_help_units=on  help='Filter time constant for a decreasing ETC Request signal.'  units='sec'  use_header_enum=off  row_header_enum={}  col_header_enum={}  use_min_max=off  min_val=-inf  max_val=inf  use_precision=off  precision=''  gain=1  offset=0  exp=1  use_mototune_group=on  mototune_group=motohawk_vardec_path(gcb)
  motohawk_delta_time : MotoHawk_lib/Extra Development Blocks/motohawk_delta_time  samp_time=-1  init_val=0  mode=Seconds (double)
  motohawk_interpolation_1d1 : MotoHawk_lib/Lookup Tables/motohawk_interpolation_1d  nam='ETCReqRiseRate'  table_data=[1:9]  show_more=on  data_type=Inherit from 'Table Data'  storage=NonAdaptive  read_level=1  write_level=1  ovr_cals=on  use_help=on  help='Limits rise rate of ETCRequestFiltered.'  units='%/sec'  use_min_max=on  min_val=0  max_val=10000  use_precision=on  precision=''  gain=1  offset=0  exp=1  use_links=off  prelookup_block=''  output_name=''  use_mototune_group=on  mototune_group=motohawk_vardec_path(gcb)
  motohawk_interpolation_1d3 : MotoHawk_lib/Lookup Tables/motohawk_interpolation_1d  nam='ETCReqFallRate'  table_data=[1:9]  show_more=on  data_type=Inherit from 'Table Data'  storage=NonAdaptive  read_level=1  write_level=1  ovr_cals=on  use_help=on  help='Limits fall rate of ETCRequestFiltered.'  units='%/sec'  use_min_max=on  min_val=-10000  max_val=0  use_precision=on  precision=''  gain=1  offset=0  exp=1  use_links=off  prelookup_block=''  output_name=''  use_mototune_group=on  mototune_group=motohawk_vardec_path(gcb)
  motohawk_interpolation_2d : MotoHawk_lib/Lookup Tables/motohawk_interpolation_2d  nam='ETCRequest'  table_data=ones(17,17)  show_more=on  data_type=Inherit from 'Table Data'  storage=NonAdaptive  read_level=1  write_level=1  ovr_cals=on  use_help=on  help='Driver demand table'  units='%'  use_min_max=on  min_val=0  max_val=100  use_precision=off  precision=''  gain=1  offset=0  exp=1  use_links=off  row_prelookup_block=''  col_prelookup_block=''  output_name=''  use_mototune_group=off  mototune_group=motohawk_vardec_path(gcb)
  motohawk_prelookup : MotoHawk_lib/Lookup Tables/motohawk_prelookup  nam='APP17'  breakpoint_data=[0 5 10 15 20 25 30 35 40 45 50 55 60 65 70 75 80]  show_more=on  data_type=Inherit from 'Table Data'  storage=Constant  read_level=1  write_level=1  ovr_cals=on  use_help=on  help='Index of APP for driver demand'  units='%'  use_min_max=on  min_val=0  max_val=100  use_precision=on  precision=''  gain=1  offset=0  exp=1  use_links=off  input_name=''  use_mototune_group=on  mototune_group=motohawk_vardec_path(gcb)
  motohawk_probe : MotoHawk_lib/Calibration & Probing Blocks/motohawk_probe  nam='ETCReqFilterConst'  show_more=on  name_source=Use Parameter  read_level=1  view_as=Number  enum_struct={'Disabled', 'Enabled'}  vector_style=Wide Row  use_help_units=off  help=''  units=''  use_header_enum=off  row_header_enum={}  col_header_enum={}  use_precision=off  precision=''  gain=1  offset=0  exp=1  use_mototune_group=on  mototune_group=motohawk_vardec_path(gcb)
  motohawk_probe1 : MotoHawk_lib/Calibration & Probing Blocks/motohawk_probe  nam='FilteredETCRequest'  show_more=on  name_source=Use Parameter  read_level=1  view_as=Number  enum_struct={'Disabled', 'Enabled'}  vector_style=Wide Row  use_help_units=on  help='Final ETC request'  units='%'  use_header_enum=off  row_header_enum={}  col_header_enum={}  use_precision=off  precision=''  gain=1  offset=0  exp=1  use_mototune_group=on  mototune_group=motohawk_vardec_path(gcb)
  motohawk_probe2 : MotoHawk_lib/Calibration & Probing Blocks/motohawk_probe  nam='ETCRequestDirection'  show_more=on  name_source=Use Parameter  read_level=1  view_as=Enumeration  enum_struct={'Decreasing', 'Increasing'}  vector_style=Wide Row  use_help_units=on  help=''  units=''  use_header_enum=off  row_header_enum={}  col_header_enum={}  use_precision=off  precision=''  gain=1  offset=0  exp=1  use_mototune_group=on  mototune_group=motohawk_vardec_path(gcb)
  ETCReqFilt : Outport
  ETCReqRaw : Outport  Port=2
  APP Idx : Outport  Port=3
  wires:
  motohawk_prelookup/1 -> APP Idx/1, motohawk_interpolation_2d/2
  APP Pcnt/1 -> motohawk_prelookup/1
  motohawk_interpolation_2d/1 -> Relational Operator3/2, Relational Operator2/2, First Order Low Pass/1, ETCReqRaw/1, Unit Delay4/1
  PassThrough1/1(Out1) -> Merge/1
  PassThrough2/1(Out1) -> Merge/2
  Relational Operator2/1 -> PassThrough2/Enable
  Relational Operator3/1 -> PassThrough1/Enable, motohawk_probe2/1
  Merge/1 -> MinMax/2, motohawk_probe/1
  MinMax/1 -> Product/2
  motohawk_delta_time/1 -> MinMax/1, Product/1
  Product/1 -> First Order Low Pass/2
  Unit Delay2/1 -> Relational Operator2/1, Relational Operator3/1
  Unit Delay1/1 -> Unit Delay2/1
  Unit Delay3/1 -> Unit Delay1/1
  Unit Delay4/1 -> Unit Delay3/1
  Variable Rate Limiter/1(output) -> ETCReqFilt/1, motohawk_probe1/1
  motohawk_interpolation_1d1/1 -> Variable Rate Limiter/2(rise rate)
  motohawk_interpolation_1d3/1 -> Variable Rate Limiter/3(fall rate)
  TPS_Idx/1 -> motohawk_interpolation_1d1/1, motohawk_interpolation_1d3/1
  First Order Low Pass/1 -> Variable Rate Limiter/1(input)
  motohawk_calibration2/1 -> PassThrough2/1(In1)
  motohawk_calibration1/1 -> PassThrough1/1(In1)
  VSPD17Idx/1 -> motohawk_interpolation_2d/1
